simulink subsystem "model_procesu_1"  (R2024b)
settings: Solver=VariableStepAuto  StartTime=0.0  StopTime=10.0  RelTol=1e-3
values from neighbouring files (symbols this model uses):
  B = 1.8*B    [wykresy_regulator_calkowy.m]
settings Model: Creator=mparadow  LastModifiedBy=mparadow

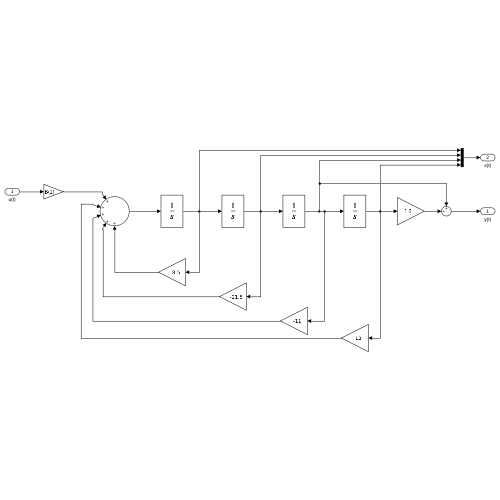
[thumbnail: Simulink's stored preview of the top-level diagram]
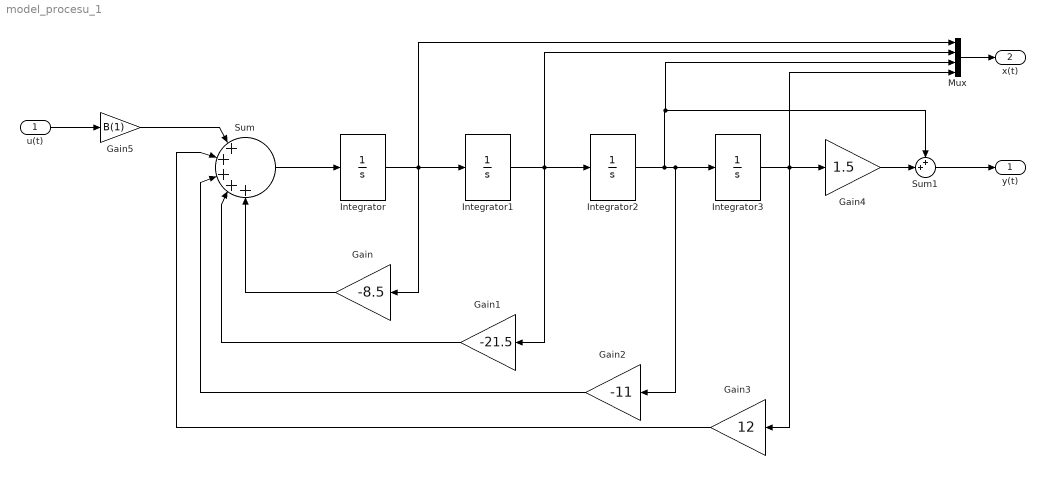
== system model_procesu_1 ==
  u(t) : Inport
  Gain : Gain  Gain=-8.5
  Gain1 : Gain  Gain=-21.5
  Gain2 : Gain  Gain=-11
  Gain3 : Gain  Gain=12
  Gain4 : Gain  Gain=1.5
  Gain5 : Gain  Gain=B(1)
  Integrator : Integrator  InitialCondition=-4
  Integrator1 : Integrator  InitialCondition=-2
  Integrator2 : Integrator  InitialCondition=-2
  Integrator3 : Integrator  InitialCondition=-1
  Mux : Mux
  Sum : Sum  Inputs=|+++++
  Sum1 : Sum  Inputs=++|
  y(t) : Outport
  x(t) : Outport  Port=2
  wires:
  Sum/1 -> Integrator/1
  Integrator/1 -> Gain/1, Integrator1/1, Mux/1
  Integrator1/1 -> Gain1/1, Integrator2/1, Mux/2
  Integrator2/1 -> Sum1/1, Mux/3, Gain2/1, Integrator3/1
  Gain4/1 -> Sum1/2
  Integrator3/1 -> Gain3/1, Gain4/1, Mux/4
  Sum1/1 -> y(t)/1
  Gain/1 -> Sum/5
  Gain1/1 -> Sum/4
  Gain2/1 -> Sum/3
  Gain3/1 -> Sum/2
  Mux/1 -> x(t)/1
  u(t)/1 -> Gain5/1
  Gain5/1 -> Sum/1
